simulink model "C2_Wideband_Filter"  (R2019b)
settings: Solver=FixedStepAuto  StartTime=0.0  StopTime=testtime  RelTol=1e-3
InitFcn:
  | AN_InitFcn_Callback
StopFcn:
  | AN_StopFcn_Callback
undefined symbols (not defined in the file or in its folder): cf, dfilt, norm_gainc2
libraries: dsparch4 x1
settings Model: Creator=mblun  LastModifiedBy=cb50701
settings DataIOCC: SaveOutput=off  SaveTime=off
settings OptimizationCC: BlockReduction=off  ConditionallyExecuteInputs=off  DefaultParameterBehavior=Inlined
settings SFSimCC: CustomCodeUndefinedFunction=UseInterfaceOnly
settings RTWCC: GenerateReport=on

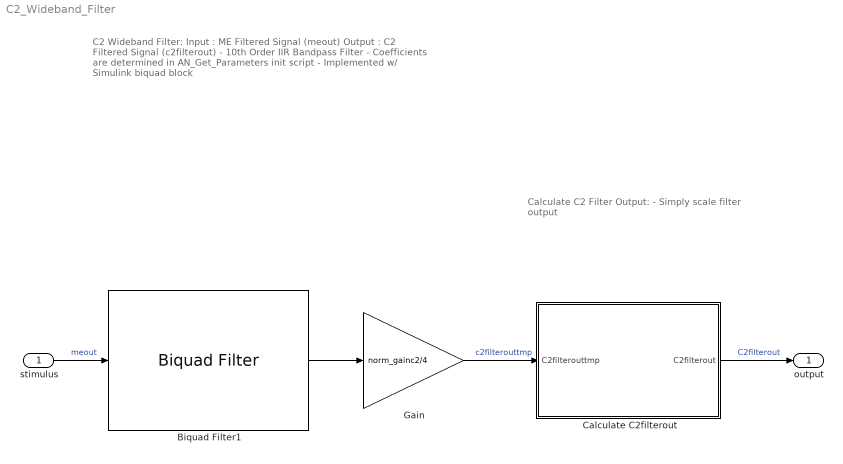
== system C2_Wideband_Filter ==
  note: C2 Wideband Filter:
      |
      | Input : ME Filtered Signal (meout)
      |
      | Output : C2 Filtered Signal (c2filterout)
      |
      | - 10th Order IIR Bandpass Filter
      |
      | - Coefficients are determined in AN_Get_Parameters init script
      |
      | - Implemented w/ Simulink biquad block
  note: Calculate C2 Filter Output:
      |
      | - Simply scale filter output
  stimulus : Inport  OutDataTypeStr=double  PortDimensions=[1 1]  SampleTime=[2.0833333333333333e-05,0]
  Biquad Filter1 : dsparch4/Biquad Filter  FilterSource=Dialog parameters  CoeffSource=Specify via dialog  FilterObject=dfilt.df2tsos([1 0.3 0.4],[1 0.1 0.2])  IIRFiltStruct=Direct form II transposed  BiQuadCoeffs=C2coeffs  ScaleValues=1  IC=0  ICnum=0  ICden=0  a0Flag=Warning  optimizeScaleValues=on  ScaleValueMode=Specify via input port (g)  roundingMode=Floor  overflowMode=on  scaleValueFracLength=14  denProdOutputFracLength=30  denAccumFracLength=30  secondMemoryFracLength=15
      settings: SourceProductName=DSP System Toolbox
  Calculate C2filterout : Subsystem
  Gain : Gain  Gain=norm_gainc2/4
  output : Outport  OutDataTypeStr=double  PortDimensions=[1 1]  SampleTime=[2.0833333333333333e-05,0]  VectorParamsAs1DForOutWhenUnconnected=off
  wires:
  stimulus/1 -> Biquad Filter1/1  "meout"
  Biquad Filter1/1 -> Gain/1
  Gain/1 -> Calculate C2filterout/1(C2filterouttmp)  "c2filterouttmp"
  Calculate C2filterout/1(C2filterout) -> output/1  "C2filterout"

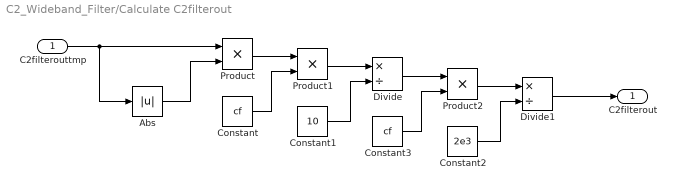
== system C2_Wideband_Filter/Calculate C2filterout ==
  C2filterouttmp : Inport
  Abs : Abs
  Constant : Constant  Value=cf  SampleTime=-1
  Constant1 : Constant  Value=10  SampleTime=-1
  Constant2 : Constant  Value=2e3  SampleTime=-1
  Constant3 : Constant  Value=cf  SampleTime=-1
  Divide : Product  Inputs=*/  SaturateOnIntegerOverflow=on  RndMeth=Zero
  Divide1 : Product  Inputs=*/  SaturateOnIntegerOverflow=on  RndMeth=Zero
  Product : Product
  Product1 : Product
  Product2 : Product
  C2filterout : Outport  VectorParamsAs1DForOutWhenUnconnected=off
  wires:
  Divide1/1 -> C2filterout/1
  Divide/1 -> Product2/1
  Constant3/1 -> Product2/2
  Constant2/1 -> Divide1/2
  Product2/1 -> Divide1/1
  Constant1/1 -> Divide/2
  Product1/1 -> Divide/1
  Constant/1 -> Product1/2
  Product/1 -> Product1/1
  Abs/1 -> Product/2
  C2filterouttmp/1 -> Abs/1, Product/1
